simulink model "linTest"  (R2024a)
settings: Solver=VariableStepAuto  StartTime=0.0  StopTime=200  RelTol=1e-3
values from neighbouring files (symbols this model uses):
  Kpi = lqr(sys, Q, R)    [QRerr_LQI.m]    (also in alexisignoringme8.mat = [9.62344892608e-17 -1.21933000029e-16 1.4312558077e-15 29.45)
  Xe = X(:,idx(2)+1)    [QRerr_LQI.m]    (also in QRerr_p.m; alexisignoringme4.mat = [24.9726490597 0 -1.16896704065 0 0 0 -8.24889531393e-07 -0.; alexisignoringme5.mat = [24.9726490597 0 -1.16896704065 0 0 0 -8.24889531393e-07 0.0; alexisignoringme6.mat = [24.9726490597 0 -1.16896704065 0 0 0 -8.24889531393e-07 0.0)
  Xes = X(:,idx(2))    [QRerr_LQI.m]    (also in QRerr_p.m; alexisignoringme4.mat = [0.00351658839646 0 -9.99999599468 0 0 0 2.7327442949e-09 -4; alexisignoringme5.mat = [0 0 -1.11199998303 0 0 0 -1.38069247376e-09 1.48137256273e-; alexisignoringme6.mat = [0 0 -1.11199998303 0 0 0 -1.38069247376e-09 1.48137256273e-)
undefined symbols (not defined in the file or in its folder): sys_a
settings Model: Creator=Jem  LastModifiedBy=Jem

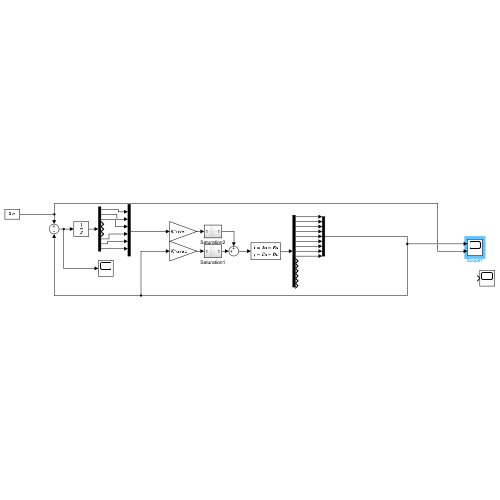
[thumbnail: Simulink's stored preview of the top-level diagram]
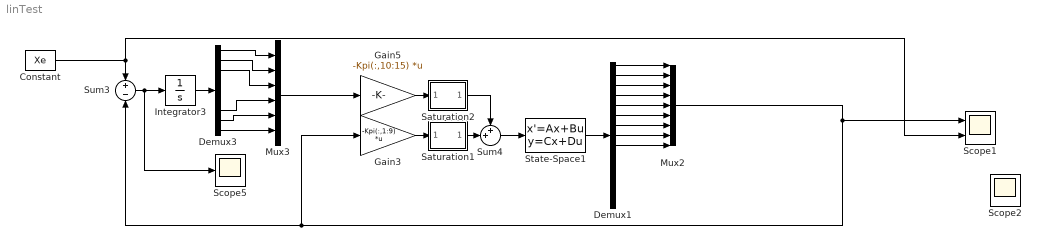
== system linTest ==
  Constant : Constant  Value=Xe
  Demux1 : Demux  Outputs=15
  Demux3 : Demux  Outputs=9
  Gain3 : Gain  Gain=-Kpi(:,1:9)  Multiplication=Matrix(K*u) (u vector)
  Gain5 : Gain  Gain=-Kpi(:,10:15)  Multiplication=Matrix(K*u) (u vector)
  Integrator3 : Integrator
  Mux2 : Mux  Inputs=9
  Mux3 : Mux  Inputs=6
  Saturation1 : Subsystem
  Saturation2 : Subsystem
  Scope1 : Scope  NumInputPorts=2
  Scope2 : Scope
  Scope5 : Scope
  State-Space1 : StateSpace  A=sys_a.A  B=sys_a.B  C=sys_a.C  D=sys_a.D  InitialCondition=[Xes; 0; 0; 0; 0; 0; 0]
  Sum3 : Sum  Inputs=+-
  Sum4 : Sum  Inputs=++|
  wires:
  State-Space1/1 -> Demux1/1
  Mux2/1 -> Scope1/1, Gain3/1, Sum3/2
  Constant/1 -> Sum3/1, Scope1/2
  Gain3/1 -> Saturation1/1(In1)
  Demux1/1 -> Mux2/1
  Demux1/2 -> Mux2/2
  Demux1/3 -> Mux2/3
  Demux1/4 -> Mux2/4
  Demux1/5 -> Mux2/5
  Demux1/6 -> Mux2/6
  Demux1/7 -> Mux2/7
  Demux1/8 -> Mux2/8
  Demux1/9 -> Mux2/9
  Sum4/1 -> State-Space1/1
  Sum3/1 -> Scope5/1, Integrator3/1
  Integrator3/1 -> Demux3/1
  Demux3/1 -> Mux3/1
  Demux3/2 -> Mux3/2
  Demux3/3 -> Mux3/3
  Demux3/7 -> Mux3/4
  Demux3/8 -> Mux3/5
  Demux3/9 -> Mux3/6
  Mux3/1 -> Gain5/1
  Gain5/1 -> Saturation2/1(In1)
  Saturation1/1(Out1) -> Sum4/2
  Saturation2/1(Out1) -> Sum4/1

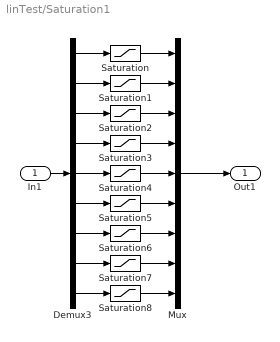
== system linTest/Saturation1 ==
  In1 : Inport
  Demux3 : Demux  Outputs=9
  Mux : Mux  Inputs=9
  Saturation : Saturate
  Saturation1 : Saturate
  Saturation2 : Saturate
  Saturation3 : Saturate  UpperLimit=1.6*150*9.81  LowerLimit=-1000
  Saturation4 : Saturate  UpperLimit=1.6*150*9.81  LowerLimit=-1000
  Saturation5 : Saturate  UpperLimit=1.6*150*9.81  LowerLimit=-1000
  Saturation6 : Saturate  UpperLimit=700  LowerLimit=-700
  Saturation7 : Saturate  UpperLimit=700  LowerLimit=-700
  Saturation8 : Saturate  UpperLimit=700  LowerLimit=-700
  Out1 : Outport
  wires:
  Demux3/9 -> Saturation8/1
  Saturation8/1 -> Mux/9
  Demux3/8 -> Saturation7/1
  Saturation7/1 -> Mux/8
  Demux3/7 -> Saturation6/1
  Saturation6/1 -> Mux/7
  Demux3/6 -> Saturation5/1
  Saturation5/1 -> Mux/6
  Saturation4/1 -> Mux/5
  Demux3/5 -> Saturation4/1
  Saturation3/1 -> Mux/4
  Demux3/4 -> Saturation3/1
  Demux3/3 -> Saturation2/1
  Saturation2/1 -> Mux/3
  Demux3/2 -> Saturation1/1
  Saturation1/1 -> Mux/2
  Saturation/1 -> Mux/1
  Demux3/1 -> Saturation/1
  Mux/1 -> Out1/1
  In1/1 -> Demux3/1

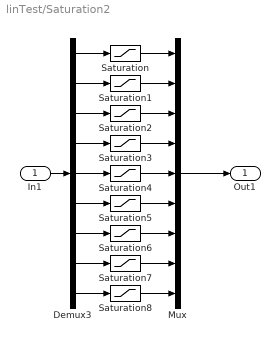
== system linTest/Saturation2 ==
  In1 : Inport
  Demux3 : Demux  Outputs=9
  Mux : Mux  Inputs=9
  Saturation : Saturate
  Saturation1 : Saturate
  Saturation2 : Saturate
  Saturation3 : Saturate  UpperLimit=1.6*150*9.81  LowerLimit=-1000
  Saturation4 : Saturate  UpperLimit=1.6*150*9.81  LowerLimit=-1000
  Saturation5 : Saturate  UpperLimit=1.6*150*9.81  LowerLimit=-1000
  Saturation6 : Saturate  UpperLimit=700  LowerLimit=-700
  Saturation7 : Saturate  UpperLimit=700  LowerLimit=-700
  Saturation8 : Saturate  UpperLimit=700  LowerLimit=-700
  Out1 : Outport
  wires:
  In1/1 -> Demux3/1
  Mux/1 -> Out1/1
  Demux3/1 -> Saturation/1
  Saturation/1 -> Mux/1
  Saturation1/1 -> Mux/2
  Demux3/2 -> Saturation1/1
  Saturation2/1 -> Mux/3
  Demux3/3 -> Saturation2/1
  Demux3/4 -> Saturation3/1
  Saturation3/1 -> Mux/4
  Demux3/5 -> Saturation4/1
  Saturation4/1 -> Mux/5
  Saturation5/1 -> Mux/6
  Demux3/6 -> Saturation5/1
  Saturation6/1 -> Mux/7
  Demux3/7 -> Saturation6/1
  Saturation7/1 -> Mux/8
  Demux3/8 -> Saturation7/1
  Saturation8/1 -> Mux/9
  Demux3/9 -> Saturation8/1
